simulink model "power_3phPWM_modified"  (Simulink 7.5)
settings: Solver=FixedStepDiscrete  SolverMode=SingleTasking  StartTime=0.0  StopTime=0.1  FixedStep=Ts  RelTol=1e-3
InitFcn:
  | Ts=1/60/3240;
undefined symbols (not defined in the file or in its folder): D1, Delta
libraries: powerlib x8, powerlib_extras x1
Description:
  | Copyright 2008-2009 The MathWorks(TM), Inc.
settings Model: Creator=patrice  LastModifiedBy=IS  ExtModeTrigMode=oneshot  ExtModeArmWhenConnect=off  ExtModeAutoUpdateStatusClock=off
settings DataIOCC: LimitDataPoints=off  SignalLoggingName=sigsOut
settings OptimizationCC: BlockReduction=off  BooleanDataType=off  InlineInvariantSignals=on  InitFltsAndDblsToZero=on
settings DebuggingCC: SaveWithParameterizedLinksMsg=none  CheckExecutionContextPreStartOutputMsg=on  CheckExecutionContextRuntimeOutputMsg=on  SignalResolutionControl=TryResolveAllWithWarning  SolverPrmCheckMsg=none  MultiTaskDSMMsg=warning  MultiTaskCondExecSysMsg=none  StrictBusMsg=None
settings HardwareCC: TargetUnknown=on
settings RTWCC: IncludeERTFirstTime=on
settings GRTTargetCC: TargetFcnLib=ansi_tfl_tmw.mat

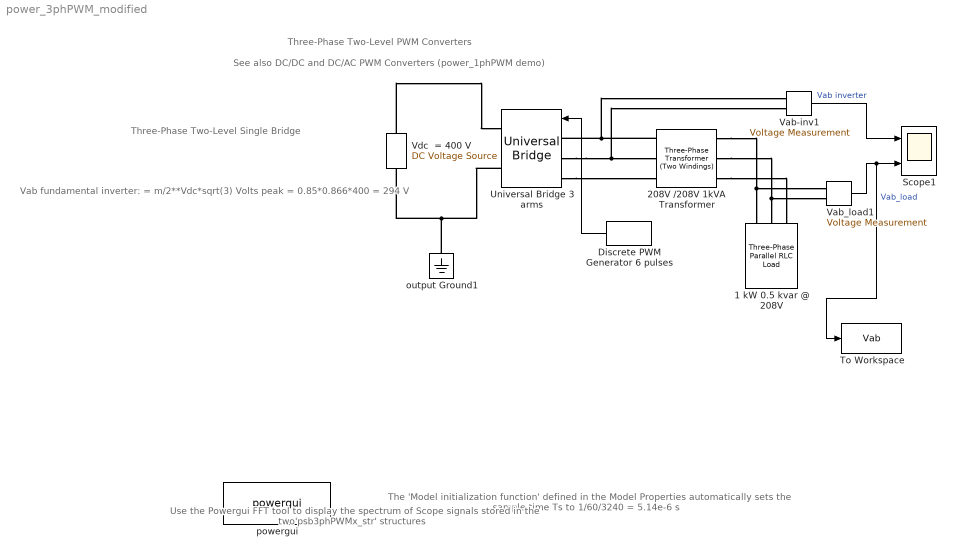
== system power_3phPWM_modified ==
  note: Three-Phase Two-Level PWM Converters
  note: See also DC/DC and DC/AC PWM Converters (power_1phPWM demo)
  note: Vab fundamental inverter:
      | = m/2**Vdc*sqrt(3) Volts peak
      | = 0.85*0.866*400
      | = 294 V
  note: Three-Phase Two-Level
      | Single Bridge
  note: The 'Model  initialization function' defined in the
      | Model Properties automatically sets the sample time Ts
      | to 1/60/3240 = 5.14e-6 s
  note: Use the Powergui FFT tool to display the
      | spectrum of Scope signals stored in the
      | two'psb3phPWMx_str' structures
  1 kW 0.5 kvar @ 208V : powerlib/Elements/Three-Phase Parallel RLC Load  DialogController=POWERSYS.PowerSysDialog  PhysicalDomain=powersysdomain  SubClassName=unknown  LeftPortType=p1  RightPortType=p1  LConnTagsString=A|B|C  Configuration=Y (grounded)  NominalVoltage=208  NominalFrequency=60  ActivePower=1000  InductivePower=0  CapacitivePower=500  Measurements=None
  208V /208V 1kVA Transformer : powerlib/Elements/Three-Phase Transformer (Two Windings)  DialogController=POWERSYS.PowerSysDialog  SystemSampleTime=-1  Winding1Connection=Delta (D1)  UNITS=pu  NominalPower=[ 1000 , 60 ]  Winding1=[ 208 , 0.002 , 0.04 ]  Winding2Connection=Yg  Winding2=[ 208 , 0.002 , 0.04 ]  SetSaturation=off  Rm=200  Lm=200  Saturation="[ 0,0  ;  0.005,1.2  ;  1.0,1.4 ]"  Hysteresis=off  DataFile='hysteresis'  SetInitialFlux=off  InitialFluxes=[ 0.8 , -0.8 , 0.7 ]  Measurements=None  MoreParameters=off  BreakLoop=off  DataType=off  TransfoNumber=0
  Discrete PWM Generator 6 pulses : powerlib_extras/Discrete  Control Blocks/Discrete PWM Generator  DialogController=POWERSYS.PowerSysDialog  SystemSampleTime=-1  GeneratorMode="3-arm  bridge (6 pulses)"  Fc=1080  Ts=Ts  Internal=on  mIndex=0.85  Freq=60  Phase=0
  Scope1 : Scope  NumInputPorts=2
      settings: TimeRange=0.1  YMin=-500~-400  YMax=500~500  SaveName=psb3phPWM1_str  MaxDataPoints=500000
  To Workspace : ToWorkspace  VariableName=Vab  SampleTime=-1  SaveFormat=Array
  Universal Bridge 3 arms : powerlib/Power Electronics/Universal Bridge  DialogController=POWERSYS.PowerSysDialog  SystemSampleTime=-1  Arms=3  SnubberResistance=10000  SnubberCapacitance=inf  Device=IGBT / Diodes  Ron=1e-4  Lon=0  ForwardVoltages="[  1  1  ]"  ForwardVoltage=.8  GTOparameters=[ 10e-6 , 20e-6 ]  IGBTparameters=[ 1e-6 , 2e-6 ]  Measurements=None  Measurements_2=None  converterType=Rectifier
  Vab-inv1 : powerlib/Measurements/Voltage Measurement  Tag=PoWeRsYsTeMmEaSuReMeNt  DialogController=POWERSYS.PowerSysDialog  SystemSampleTime=-1  PhasorSimulation=off  OutputType=Magnitude  PSBequivalent=0
  Vab_load1 : powerlib/Measurements/Voltage Measurement  Tag=PoWeRsYsTeMmEaSuReMeNt  DialogController=POWERSYS.PowerSysDialog  SystemSampleTime=-1  PhasorSimulation=off  OutputType=Magnitude  PSBequivalent=0
  Vdc  = 400 V : powerlib/Electrical Sources/DC Voltage Source  Description=source block  DialogController=POWERSYS.PowerSysDialog  SystemSampleTime=-1  Amplitude=400  Measurements=None
      settings: AttributesFormatString=\n
  output Ground1 : powerlib/Elements/Ground  DialogController=POWERSYS.PowerSysDialog  PhysicalDomain=powersysdomain  SubClassName=unknown  LeftPortType=p1  RightPortType=p1  LConnTagsString=a
  powergui : powerlib/powergui  Priority=2  SystemSampleTime=-1  SimulationMode=Discrete  SampleTime=Ts  frequency=60  SPID=off  DisableSnubberDevices=off  DisableRonSwitches=off  DisableVfSwitches=off  SwTol=0  Interpol=off  frequencyindice=0  echomessages=on  HookPort=off  DisplayEquations=off  FunctionMessages=off  EnableUseOfTLC=off  x0status=blocks  RestoreLinks=warning  ResistiveCurrentMeasurement=off  Frange=[0:2:500]  Ylog=off  Xlog=off  ShowGrid=off  save=off  variable=ZData  structure=psb3phPWM1_str  ZoomFFT=off  StartTime=0.1 - 2/60  cycles=2  DisplayStyle=1  fundamental=60  FreqAxis=on  MaxFrequency=2400  frequencyindicesteady=1  RmsSteady=1  display=off  Ts=0  methode=off
  wires:
  Discrete PWM Generator 6 pulses/1 -> Universal Bridge 3 arms/1
  Vab_load1/1 -> Scope1/2, To Workspace/1  "Vab_load"
  Vab-inv1/1 -> Scope1/1  "Vab inverter"
  connections:
  Universal Bridge 3 arms/LConn2 -- Vab-inv1/LConn2 -- 208V /208V 1kVA Transformer/LConn2
  Universal Bridge 3 arms/LConn3 -- 208V /208V 1kVA Transformer/LConn3
  208V /208V 1kVA Transformer/RConn3 -- 1 kW 0.5 kvar @ 208V/LConn3
  208V /208V 1kVA Transformer/RConn1 -- 1 kW 0.5 kvar @ 208V/LConn1 -- Vab_load1/LConn1
  208V /208V 1kVA Transformer/RConn2 -- 1 kW 0.5 kvar @ 208V/LConn2 -- Vab_load1/LConn2
  output Ground1/LConn1 -- Vdc  = 400 V/LConn1 -- Universal Bridge 3 arms/RConn2
  Vdc  = 400 V/RConn1 -- Universal Bridge 3 arms/RConn1
  208V /208V 1kVA Transformer/LConn1 -- Universal Bridge 3 arms/LConn1 -- Vab-inv1/LConn1
